simulink model "dt_system"  (R2022a)
settings: Solver=ode45  StartTime=0.0  StopTime=tfinal  FixedStep=T  MaxStep=0.01  RelTol=1e-12  AbsTol=1e-12  EnableMultiTasking=on
values from neighbouring files (symbols this model uses):
  D_dem = dd    [question1.m]    (also in question2.m)
  D_num = nd    [question1.m]    (also in question2.m)
  G_dem = a    [question1.m]    (also in question2.m)
  G_num = b    [question1.m]    (also in question2.m)
  step_amp = 1    [question1.m]    (also in question2.m)
settings Model: Creator=cnielsen  LastModifiedBy=urban
settings SolverCC: AutoScaleAbsTol=off  AlgebraicLoopSolver=TrustRegion
settings DataIOCC: SaveFormat=Array  SignalLoggingSaveFormat=ModelDataLogs  SaveOutput=off  SaveTime=off  ReturnWorkspaceOutputs=off  Refine=5
settings OptimizationCC: ExpressionDepthLimit=2147483647  LifeSpan=inf
settings DebuggingCC: UnderspecifiedInitializationDetection=Classic  MergeDetectMultiDrivingBlocksExec=none  SolverPrmCheckMsg=warning  FcnCallInpInsideContextMsg=warning  UnconnectedInputMsg=warning  UnconnectedOutputMsg=warning  UnconnectedLineMsg=warning  StateNameClashWarn=warning  SFUnexpectedBacktrackingDiag=warning  SFNoUnconditionalDefaultTransitionDiag=warning  SFExecutionAtInitializationDiag=none  SFMachineParentedDataDiag=warning  ArithmeticOperatorsInVariantConditions=warning
settings HardwareCC: ProdBitPerPointer=32  ProdBitPerSizeT=32  ProdBitPerPtrDiffT=32  ProdLargestAtomicFloat=None  ProdIntDivRoundTo=Undefined  ProdEndianess=Unspecified  ProdWordSize=32  ProdHWDeviceType=32-bit Generic
settings ModelReferenceCC: PropagateSignalLabelsOutOfModel=off
settings SFSimCC: SimUseLocalCustomCode=off  CustomCodeUndefinedFunction=UseInterfaceOnly
settings RTWCC: RTWUseLocalCustomCode=off  DLArmComputeVersion=19.05
settings CodeAppCC: StateflowObjectComments=on
settings GRTTargetCC: TargetLangStandard=C89/C90 (ANSI)  CombineOutputUpdateFcns=off  GRTInterface=on
settings ConfigComp: CovMetricSettings=dw  CovSaveCumulativeToWorkspaceVar=on  CovSaveSingleToWorkspaceVar=on  CovExternalEMLEnable=off

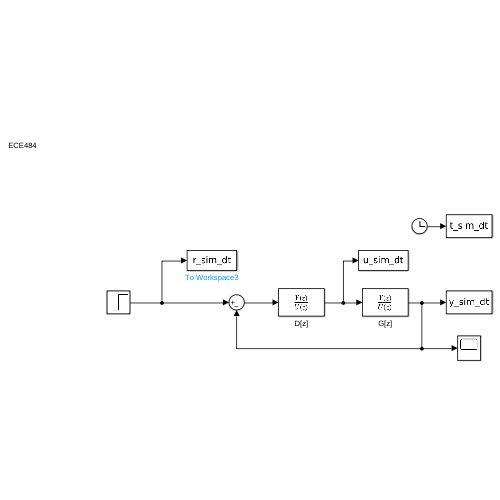
[thumbnail: Simulink's stored preview of the top-level diagram]
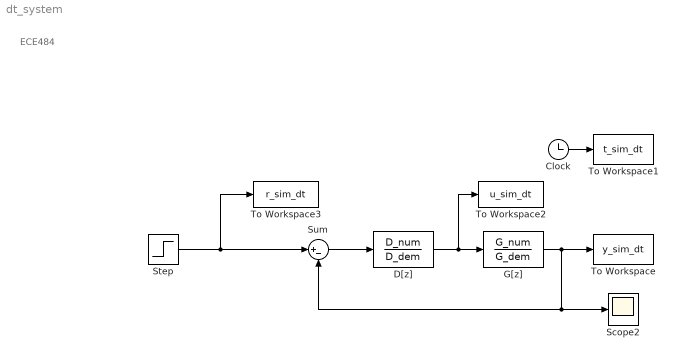
== system dt_system ==
  note: ECE484
  Clock : Clock
  D[z] : DiscreteTransferFcn  Numerator=D_num  Denominator=D_dem
  G[z] : DiscreteTransferFcn  Numerator=G_num  Denominator=G_dem
  Scope2 : Scope
  Step : Step  Time=0  After=step_amp  SampleTime=0
  Sum : Sum  Inputs=|+-
  To Workspace : ToWorkspace  VariableName=y_sim_dt  SampleTime=-1
  To Workspace1 : ToWorkspace  VariableName=t_sim_dt  SampleTime=-1
  To Workspace2 : ToWorkspace  VariableName=u_sim_dt
  To Workspace3 : ToWorkspace  VariableName=r_sim_dt
  wires:
  Step/1 -> To Workspace3/1, Sum/1
  D[z]/1 -> G[z]/1, To Workspace2/1
  G[z]/1 -> To Workspace/1, Sum/2, Scope2/1
  Sum/1 -> D[z]/1
  Clock/1 -> To Workspace1/1
